simulink model "Fire_Detection_Video"  (R2023b)
settings: Solver=FixedStepAuto  StartTime=0.0  StopTime=60  RelTol=1e-3
undefined symbols (not defined in the file or in its folder): gray
libraries: dspvision x2
settings Model: Creator=Amir  LastModifiedBy=vahed
settings SolverCC: AlgebraicLoopSolver=TrustRegion
settings DataIOCC: ReturnWorkspaceOutputs=off
settings DebuggingCC: UnconnectedInputMsg=warning  UnconnectedOutputMsg=warning  UnconnectedLineMsg=warning  ArithmeticOperatorsInVariantConditions=warning
settings HardwareCC: ProdBitPerLong=64  ProdHWDeviceType=Intel->x86-64 (Linux 64)
settings ModelReferenceCC: EnableRefExpFcnMdlSchedulingChecks=on
settings SFSimCC: CustomCodeUndefinedFunction=UseInterfaceOnly
settings RTWCC: Description=Simulink Desktop Real-Time  SystemTargetFile=sldrt.tlc  TemplateMakefile=sldrt.tmf  RTWCompilerOptimization=on  DLArmComputeVersion=19.05
settings CodeAppCC: MaxIdLength=95
settings SimulinkDesktopRealTimeCC: TargetLibSuffix=_sldrt.a  TargetPreCompLibLocation=C:\MATLAB\R2023b\toolbox\sldrt\lib\win64  CodeReplacementLibrary=GNU C99 extensions

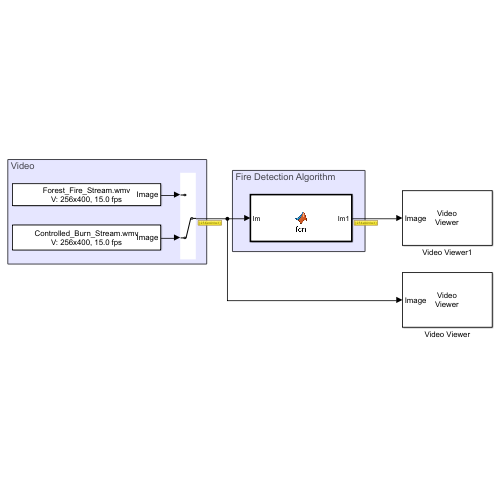
[thumbnail: Simulink's stored preview of the top-level diagram]
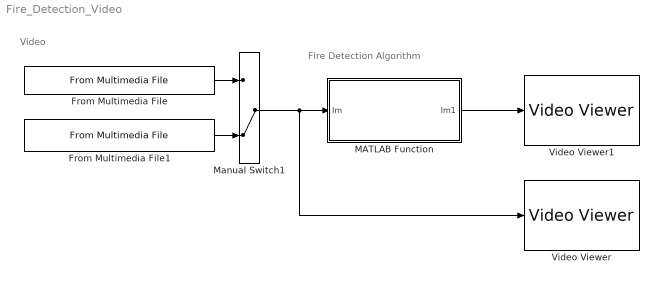
== system Fire_Detection_Video ==
  note: Fire Detection Algorithm
  note: Video
  From Multimedia File : dspvision/From Multimedia File  inputFilename=Forest_Fire_Stream.wmv  readRange=[1 Inf]  loop=on  numPlays=inf  outputStreams=Video only  videoDataType=single  audioDataType=double  inheritSampleTime=on  userDefinedSampleTime=1/30  noAudioOutput=off  isIntensityVideo=off  fourcc=RGB  colorVideoFormat=One multidimensional signal  outputEOF=off  dataOrg=Column-major  audioFrameSize=1024  computeAudioFrameSize=off  outSamplingMode=Sample based
  From Multimedia File1 : dspvision/From Multimedia File  inputFilename=Controlled_Burn_Stream.wmv  readRange=[1 Inf]  loop=on  numPlays=inf  outputStreams=Video only  videoDataType=single  audioDataType=double  inheritSampleTime=on  userDefinedSampleTime=1/30  noAudioOutput=off  isIntensityVideo=off  fourcc=RGB  colorVideoFormat=One multidimensional signal  outputEOF=off  dataOrg=Column-major  audioFrameSize=1024  computeAudioFrameSize=off  outSamplingMode=Sample based
  MATLAB Function : MATLAB Function  TreatAsAtomicUnit=on
  Manual Switch1 : ManualSwitch  CurrentSetting=0
  Video Viewer : VideoViewer  colormapValue=gray(256)  FigPos=[333.8 714 675.2 508.8]
  Video Viewer1 : VideoViewer  colormapValue=gray(256)  FigPos=[973.8 697.2 1000 528]
  wires:
  MATLAB Function/1(Im1) -> Video Viewer1/1
  Manual Switch1/1 -> Video Viewer/1, MATLAB Function/1(Im)
  From Multimedia File/1 -> Manual Switch1/1
  From Multimedia File1/1 -> Manual Switch1/2

== matlab function Fire_Detection_Video/MATLAB Function ==
  data: Im input; Im1 output
function Im1 = fcn(Im)
Im=Im.*255;
[m,n,~]=size(Im);
mask=zeros(m,n);
Im_LAB = rgb2lab(Im);
Lm=mean(mean(Im_LAB(:,:,1)));
Am=mean(mean(Im_LAB(:,:,2)));
Bm=mean(mean(Im_LAB(:,:,3)));
R_T=230;%[115 135]
for i=1:m
    for j=1:n
        if Im(i,j,1)>=R_T
            if Im(i,j,1)>=Im(i,j,2) && Im(i,j,2)>=Im(i,j,3)
                if Im(i,j,2)/(Im(i,j,1)+255)>=0.25 && Im(i,j,2)/(Im(i,j,1)+255)<=0.65
                    if Im(i,j,3)/(Im(i,j,1)+255)>=0.05 && Im(i,j,3)/(Im(i,j,1)+255)<=0.45
                        if Im(i,j,3)/(Im(i,j,2)+255)>=0.2 && Im(i,j,3)/(Im(i,j,2)+255)<=0.6
                            if Im_LAB(i,j,1)>=Lm && Im_LAB(i,j,2)>=Am && Im_LAB(i,j,3)>=Bm %&& Im_LAB(i,j,3)>=Im_LAB(i,j,2)
                                mask(i,j)=1;
                            end
                        end
                    end
                end
            end
        end
    end
end
Im1= bsxfun(@times, Im, cast(mask, 'like', Im))./255;
% Im1=mask;
